simulink model "commander"  (R2022b)
settings: Solver=FixedStepAuto  StartTime=0.0  StopTime=100  FixedStep=0.5  RelTol=1e-3
(part 1 of 3)
settings Model: DataDictionary=px4_dict.sldd  Creator=DELL  LastModifiedBy=DELL
settings OptimizationCC: DefaultParameterBehavior=Inlined  EnhancedBackFolding=on  PassReuseOutputArgsAs=Individual arguments  ZeroExternalMemoryAtStartup=off  ZeroInternalMemoryAtStartup=off  OptimizeBlockOrder=speed  DifferentSizesBufferReuse=on  OptimizationCustomize=off  EfficientTunableParamExpr=on
settings DebuggingCC: ParameterPrecisionLossMsg=none  ParameterTunabilityLossMsg=error  UnconnectedInputMsg=warning  UnconnectedOutputMsg=warning  UnconnectedLineMsg=warning  SFUnusedDataAndEventsDiag=none  UnitsInconsistencyMsg=none
settings ModelReferenceCC: EnableRefExpFcnMdlSchedulingChecks=on
settings RTWCC: Description=Embedded Coder  SystemTargetFile=ert.tlc  TemplateMakefile=ert_default_tmf  DLArmComputeVersion=19.05
settings CodeAppCC: ForceParamTrailComments=on  IgnoreCustomStorageClasses=off  OperatorAnnotations=on  SimulinkDataObjDesc=on  SFDataObjDesc=on  InsertBlockDesc=on
settings ERTTargetCC: TargetLangStandard=C99 (ISO)  GenerateSampleERTMain=on  InlinedParameterPlacement=NonHierarchical  ERTCustomFileTemplate=example_file_process.tlc

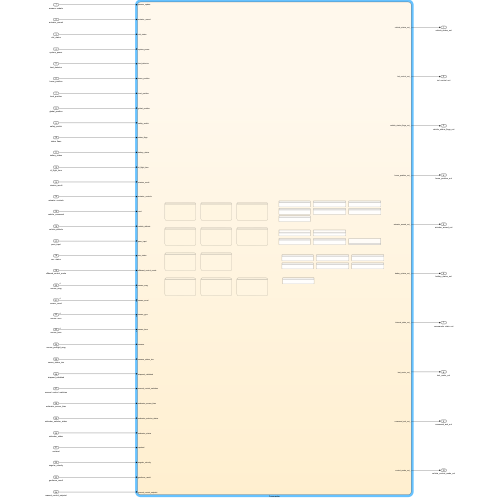
[thumbnail: Simulink's stored preview of the top-level diagram]
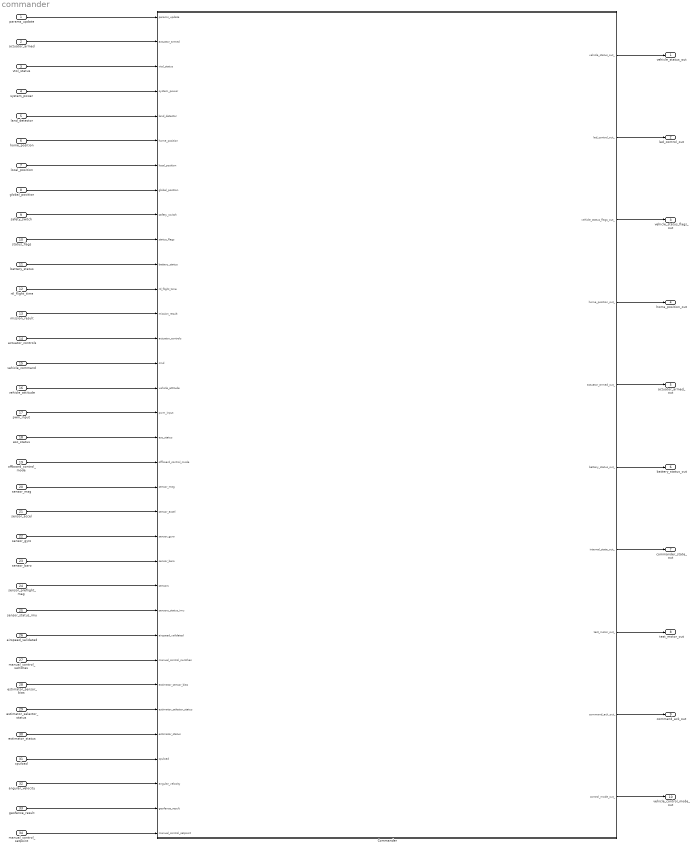
== system commander ==
  params_update : Inport  OutDataTypeStr=Bus: px4_parameter_update  BusOutputAsStruct=on
  actuator_armed : Inport  Port=2  OutDataTypeStr=Bus: px4_actuator_armed  BusOutputAsStruct=on
  vtol_status : Inport  Port=3  OutDataTypeStr=Bus: px4_vtol_vehicle_status  BusOutputAsStruct=on
  system_power : Inport  Port=4  OutDataTypeStr=Bus: px4_system_power  BusOutputAsStruct=on
  land_detector : Inport  Port=5  OutDataTypeStr=Bus: px4_vehicle_land_detected  BusOutputAsStruct=on
  home_position : Inport  Port=6  OutDataTypeStr=Bus: px4_home_position  BusOutputAsStruct=on
  local_position : Inport  Port=7  OutDataTypeStr=Bus: px4_vehicle_local_position  BusOutputAsStruct=on
  global_position : Inport  Port=8  OutDataTypeStr=Bus: px4_vehicle_global_position  BusOutputAsStruct=on
  safety_switch : Inport  Port=9  OutDataTypeStr=Bus: px4_safety  BusOutputAsStruct=on
  status_flags : Inport  Port=10  OutDataTypeStr=Bus: px4_vehicle_status_flags  BusOutputAsStruct=on
  battery_status : Inport  Port=11  OutDataTypeStr=Bus: px4_battery_status  BusOutputAsStruct=on
  rtl_flight_time : Inport  Port=12  OutDataTypeStr=Bus: px4_rtl_flight_time  BusOutputAsStruct=on
  mission_result : Inport  Port=13  OutDataTypeStr=Bus: px4_mission_result  BusOutputAsStruct=on
  actuator_controls : Inport  Port=14  OutDataTypeStr=Bus: px4_actuator_controls  BusOutputAsStruct=on
  vehicle_command : Inport  Port=15  OutDataTypeStr=Bus: px4_vehicle_command  BusOutputAsStruct=on
  vehicle_attitude : Inport  Port=16  OutDataTypeStr=Bus: px4_vehicle_attitude  BusOutputAsStruct=on
  pwm_input : Inport  Port=17  OutDataTypeStr=Bus: px4_pwm_input  BusOutputAsStruct=on
  esc_status : Inport  Port=18  OutDataTypeStr=Bus: px4_esc_status  BusOutputAsStruct=on
  offboard_control_mode : Inport  Port=19  OutDataTypeStr=Bus: px4_offboard_control_mode  BusOutputAsStruct=on
  sensor_mag : Inport  Port=20  OutDataTypeStr=Bus: px4_sensor_mag  PortDimensions=4  BusOutputAsStruct=on
  sensor_accel : Inport  Port=21  OutDataTypeStr=Bus: px4_sensor_accel  PortDimensions=4  BusOutputAsStruct=on
  sensor_gyro : Inport  Port=22  OutDataTypeStr=Bus: px4_sensor_gyro  PortDimensions=4  BusOutputAsStruct=on
  sensor_baro : Inport  Port=23  OutDataTypeStr=Bus: px4_sensor_baro  PortDimensions=4  BusOutputAsStruct=on
  sensor_preflight_mag : Inport  Port=24  OutDataTypeStr=Bus: px4_sensor_preflight_mag  LockScale=on  BusOutputAsStruct=on
  sensor_status_imu : Inport  Port=25  OutDataTypeStr=Bus: px4_sensors_status_imu  LockScale=on  BusOutputAsStruct=on
  airspeed_validated : Inport  Port=26  OutDataTypeStr=Bus: px4_airspeed_validated  LockScale=on  BusOutputAsStruct=on
  manual_control_switches : Inport  Port=27  OutDataTypeStr=Bus: px4_manual_control_switches  LockScale=on  BusOutputAsStruct=on
  estimator_sensor_bias : Inport  Port=28  OutDataTypeStr=Bus: px4_estimator_sensor_bias  LockScale=on  BusOutputAsStruct=on
  estimator_selector_status : Inport  Port=29  OutDataTypeStr=Bus: px4_estimator_selector_status  LockScale=on  BusOutputAsStruct=on
  estimator_status : Inport  Port=30  OutDataTypeStr=Bus: px4_estimator_status  LockScale=on  BusOutputAsStruct=on
  cpuload : Inport  Port=31  OutDataTypeStr=Bus: px4_cpuload  LockScale=on  BusOutputAsStruct=on
  angular_velocity : Inport  Port=32  OutDataTypeStr=Bus: px4_vehicle_angular_velocity  LockScale=on  BusOutputAsStruct=on
  geofence_result : Inport  Port=33  OutDataTypeStr=Bus: px4_geofence_result  LockScale=on  BusOutputAsStruct=on
  manual_control_setpoint : Inport  Port=34  OutDataTypeStr=Bus: px4_manual_control_setpoint  LockScale=on  BusOutputAsStruct=on
  Commander : Stateflow chart  TreatAsAtomicUnit=on
  vehicle_status_out : Outport  OutDataTypeStr=Bus: px4_vehicle_status  BusOutputAsStruct=on
  led_control_out : Outport  Port=2  OutDataTypeStr=Bus: px4_led_control  BusOutputAsStruct=on
  vehicle_status_flags_out : Outport  Port=3  OutDataTypeStr=Bus: px4_vehicle_status_flags  BusOutputAsStruct=on
  home_position_out : Outport  Port=4  OutDataTypeStr=Bus: px4_home_position  BusOutputAsStruct=on
  actuator_armed_out : Outport  Port=5  OutDataTypeStr=Bus: px4_actuator_armed  BusOutputAsStruct=on
  battery_status_out : Outport  Port=6  OutDataTypeStr=Bus: px4_battery_status  BusOutputAsStruct=on
  commander_state_out : Outport  Port=7  OutDataTypeStr=Bus: px4_commander_state  BusOutputAsStruct=on
  test_motor_out : Outport  Port=8  OutDataTypeStr=Bus: px4_test_motor  BusOutputAsStruct=on
  command_ack_out : Outport  Port=9  OutDataTypeStr=Bus: px4_vehicle_command_ack  BusOutputAsStruct=on
  vehicle_control_mode_out : Outport  Port=10  OutDataTypeStr=Bus: px4_vehicle_control_mode  BusOutputAsStruct=on
  wires:
  battery_status/1 -> Commander/11(battery_status)
  global_position/1 -> Commander/8(global_position)
  status_flags/1 -> Commander/10(status_flags)
  params_update/1 -> Commander/1(params_update)
  local_position/1 -> Commander/7(local_position)
  safety_switch/1 -> Commander/9(safety_switch)
  vtol_status/1 -> Commander/3(vtol_status)
  sensor_status_imu/1 -> Commander/25(sensors_status_imu)
  actuator_armed/1 -> Commander/2(actuator_armed)
  system_power/1 -> Commander/4(system_power)
  land_detector/1 -> Commander/5(land_detector)
  home_position/1 -> Commander/6(home_position)
  estimator_selector_status/1 -> Commander/29(estimator_selector_status)
  sensor_baro/1 -> Commander/23(sensor_baro)
  esc_status/1 -> Commander/18(esc_status)
  rtl_flight_time/1 -> Commander/12(rtl_flight_time)
  estimator_status/1 -> Commander/30(estimator_status)
  airspeed_validated/1 -> Commander/26(airspeed_validated)
  offboard_control_mode/1 -> Commander/19(offboard_control_mode)
  mission_result/1 -> Commander/13(mission_result)
  Commander/5(actuator_armed_out_) -> actuator_armed_out/1
  Commander/4(home_position_out_) -> home_position_out/1
  Commander/3(vehicle_status_flags_out_) -> vehicle_status_flags_out/1
  Commander/2(led_control_out_) -> led_control_out/1
  actuator_controls/1 -> Commander/14(actuator_controls)
  cpuload/1 -> Commander/31(cpuload)
  manual_control_switches/1 -> Commander/27(manual_control_switches)
  sensor_mag/1 -> Commander/20(sensor_mag)
  vehicle_command/1 -> Commander/15(cmd)
  vehicle_attitude/1 -> Commander/16(vehicle_attitude)
  angular_velocity/1 -> Commander/32(angular_velocity)
  estimator_sensor_bias/1 -> Commander/28(estimator_sensor_bias)
  sensor_gyro/1 -> Commander/22(sensor_gyro)
  pwm_input/1 -> Commander/17(pwm_input)
  sensor_accel/1 -> Commander/21(sensor_accel)
  sensor_preflight_mag/1 -> Commander/24(sensors)
  geofence_result/1 -> Commander/33(geofence_result)
  manual_control_setpoint/1 -> Commander/34(manual_control_setpoint)
  Commander/1(vehicle_status_out_) -> vehicle_status_out/1
  Commander/9(command_ack_out_) -> command_ack_out/1
  Commander/8(test_motor_out_) -> test_motor_out/1
  Commander/7(internal_state_out_) -> commander_state_out/1
  Commander/6(battery_status_out_) -> battery_status_out/1
  Commander/10(control_mode_out_) -> vehicle_control_mode_out/1
